simulink model "FirstItem"  (R2022b)
settings: Solver=ode4  StartTime=0.0  StopTime=45  FixedStep=0.01  RelTol=1e-3
values from neighbouring files (symbols this model uses):
  Ka = 4.5    [Item1.m]
  Kdc = 1.1    [Item1.m]
  Ki = 14.3    [Item1.m]
  Kr = -0.37    [Item1.m]
  l_MO = 80*d2r    (= 1.3962634016)    [Item1.m]
  l_TO = -2.5*d2r    (= -0.0436332312999)    [Item1.m]
  V_T = 600    [Item1.m]
  X_MO = 2000    [Item1.m]
  X_TO = 100    [Item1.m]
  Z_MO = 0    [Item1.m]
  Z_TO = 20000    [Item1.m]
libraries: simulink x1
settings Model: Creator=lagruni  LastModifiedBy=lagruni

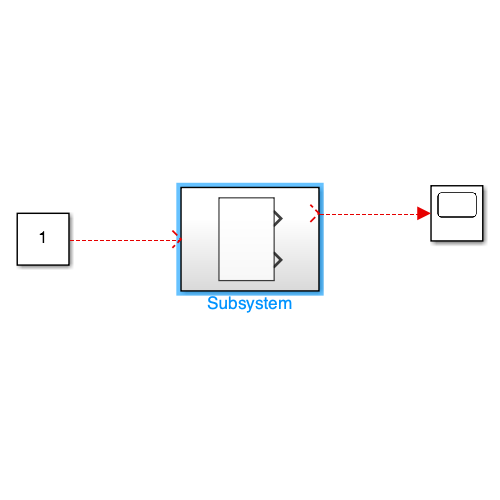
[thumbnail: Simulink's stored preview of the top-level diagram]
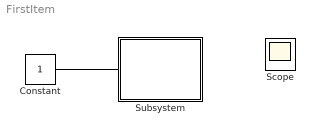
== system FirstItem ==
  Constant : Constant
  Scope : Scope
  Subsystem : Subsystem
  wires:
  Constant/1 -> ?
  ? -> Scope/1

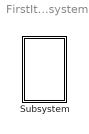
== system FirstItem/Subsystem ==
  Subsystem : Subsystem

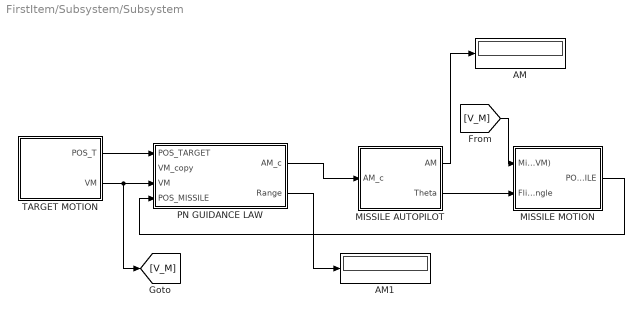
== system FirstItem/Subsystem/Subsystem ==
  AM : Display
      settings: Format=bank
  AM1 : Display
      settings: Format=bank
  MISSILE AUTOPILOT : Subsystem
  MISSILE MOTION : Subsystem
  PN GUIDANCE LAW : Subsystem
  TARGET MOTION : Subsystem
  wires:
  TARGET MOTION/1(POS_T) -> PN GUIDANCE LAW/1(POS_TARGET)
  TARGET MOTION/2(VM) -> [V_M], PN GUIDANCE LAW/3(VM)
  [V_M] -> MISSILE MOTION/1(Missile speed (VM))
  MISSILE MOTION/1(POS_MISSILE) -> PN GUIDANCE LAW/4(POS_MISSILE)
  PN GUIDANCE LAW/1(AM_c) -> MISSILE AUTOPILOT/1(AM_c)
  MISSILE AUTOPILOT/2(Theta) -> MISSILE MOTION/2(Flight path angle)
  MISSILE AUTOPILOT/1(AM) -> AM/1
  PN GUIDANCE LAW/2(Range) -> AM1/1

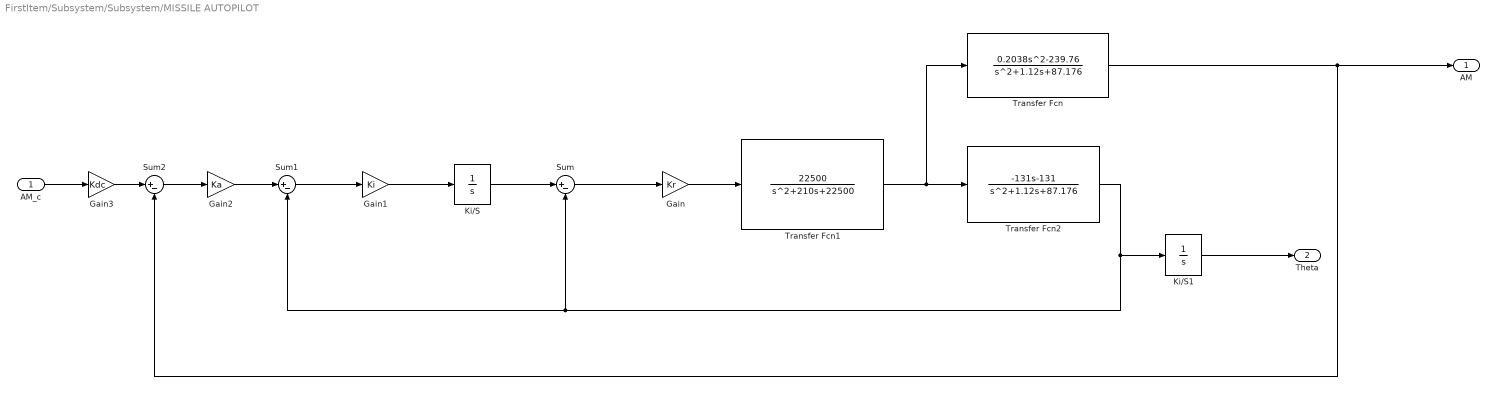
== system FirstItem/Subsystem/Subsystem/MISSILE AUTOPILOT ==
  AM_c : Inport
  Gain : Gain  Gain=Kr
  Gain1 : Gain  Gain=Ki
  Gain2 : Gain  Gain=Ka
  Gain3 : Gain  Gain=Kdc
  Ki/S : Integrator
  Ki/S1 : Integrator  InitialCondition=l_MO
  Sum : Sum  Inputs=|+-
  Sum1 : Sum  Inputs=|+-
  Sum2 : Sum  Inputs=|+-
  Transfer Fcn : TransferFcn  Numerator=[0.2038 0 -239.76]  Denominator=[1 1.12 87.176]
  Transfer Fcn1 : TransferFcn  Numerator=[22500]  Denominator=[1 210 22500]
  Transfer Fcn2 : TransferFcn  Numerator=[-131 -131]  Denominator=[1 1.12 87.176]
  AM : Outport
  Theta : Outport  Port=2
  wires:
  AM_c/1 -> Gain3/1
  Sum/1 -> Gain/1
  Transfer Fcn2/1 -> Ki/S1/1, Sum/2, Sum1/2
  Transfer Fcn1/1 -> Transfer Fcn/1, Transfer Fcn2/1
  Ki/S1/1 -> Theta/1
  Gain/1 -> Transfer Fcn1/1
  Sum1/1 -> Gain1/1
  Ki/S/1 -> Sum/1
  Gain2/1 -> Sum1/1
  Sum2/1 -> Gain2/1
  Gain3/1 -> Sum2/1
  Gain1/1 -> Ki/S/1
  Transfer Fcn/1 -> AM/1, Sum2/2

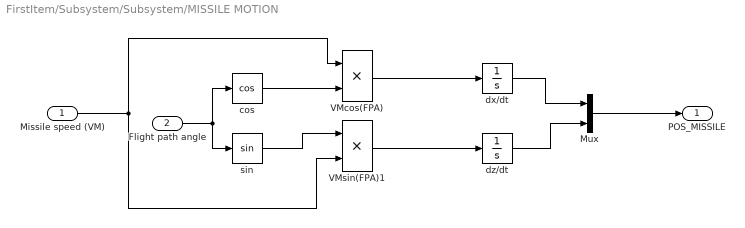
== system FirstItem/Subsystem/Subsystem/MISSILE MOTION ==
  Missile speed (VM) : Inport
  Flight path angle : Inport  Port=2
  Mux : Mux  Inputs=2
  VMcos(FPA) : Product
  VMsin(FPA)1 : Product
  cos : Trigonometry  Operator=cos
  dx/dt : Integrator  InitialCondition=X_MO
  dz/dt : Integrator  InitialCondition=Z_MO
  sin : Trigonometry
  POS_MISSILE : Outport
  wires:
  Mux/1 -> POS_MISSILE/1
  cos/1 -> VMcos(FPA)/2
  dz/dt/1 -> Mux/2
  Missile speed (VM)/1 -> VMsin(FPA)1/2, VMcos(FPA)/1
  sin/1 -> VMsin(FPA)1/1
  VMsin(FPA)1/1 -> dz/dt/1
  dx/dt/1 -> Mux/1
  VMcos(FPA)/1 -> dx/dt/1
  Flight path angle/1 -> sin/1, cos/1

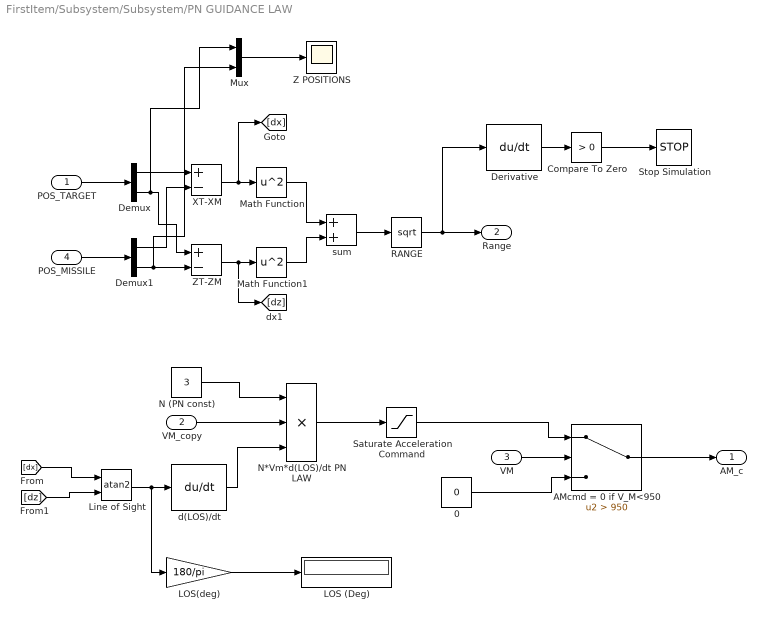
== system FirstItem/Subsystem/Subsystem/PN GUIDANCE LAW ==
  POS_TARGET : Inport
  VM_copy : Inport  Port=2
  VM : Inport  Port=3
  POS_MISSILE : Inport  Port=4
  0 : Constant  Value=0
  AMcmd = 0 if V_M<950 : Switch  Criteria=u2 > Threshold  Threshold=950  SaturateOnIntegerOverflow=off  InputSameDT=off
  Compare To Zero : simulink/Logic and Bit Operations/Compare To Zero  relop=>  OutDataTypeStr=boolean
  Demux : Demux  Outputs=2
  Demux1 : Demux  Outputs=2
  Derivative : Derivative
  LOS (Deg) : Display
  LOS(deg) : Gain  Gain=180/pi
  Line of Sight : Trigonometry  Operator=atan2
  Math Function : Math  Operator=square
  Math Function1 : Math  Operator=square
  Mux : Mux  Inputs=2
  N (PN const) : Constant  Value=3
  N*Vm*d(LOS)/dt PN LAW : Product  Inputs=3
  RANGE : Sqrt
  Saturate Acceleration Command : Saturate  UpperLimit=0  LowerLimit=-0.10
  Stop Simulation : Stop
  XT-XM : Sum  Inputs=+-
  Z POSITIONS : Scope
  ZT-ZM : Sum  Inputs=+-
  d(LOS)/dt : Derivative
  sum : Sum
  AM_c : Outport
  Range : Outport  Port=2
  wires:
  Saturate Acceleration Command/1 -> AMcmd = 0 if V_M<950/1
  LOS(deg)/1 -> LOS (Deg)/1
  RANGE/1 -> Range/1, Derivative/1
  VM_copy/1 -> N*Vm*d(LOS)/dt PN LAW/2
  POS_TARGET/1 -> Demux/1
  N (PN const)/1 -> N*Vm*d(LOS)/dt PN LAW/1
  VM/1 -> AMcmd = 0 if V_M<950/2
  AMcmd = 0 if V_M<950/1 -> AM_c/1
  POS_MISSILE/1 -> Demux1/1
  N*Vm*d(LOS)/dt PN LAW/1 -> Saturate Acceleration Command/1
  Mux/1 -> Z POSITIONS/1
  Demux1/1 -> XT-XM/2
  Math Function1/1 -> sum/2
  [dz] -> Line of Sight/2
  sum/1 -> RANGE/1
  Demux/1 -> XT-XM/1
  ZT-ZM/1 -> [dz], Math Function1/1
  0/1 -> AMcmd = 0 if V_M<950/3
  Compare To Zero/1 -> Stop Simulation/1
  Demux1/2 -> Mux/2, ZT-ZM/2
  Demux/2 -> Mux/1, ZT-ZM/1
  XT-XM/1 -> [dx], Math Function/1
  Derivative/1 -> Compare To Zero/1
  Line of Sight/1 -> LOS(deg)/1, d(LOS)/dt/1
  Math Function/1 -> sum/1
  d(LOS)/dt/1 -> N*Vm*d(LOS)/dt PN LAW/3
  [dx] -> Line of Sight/1

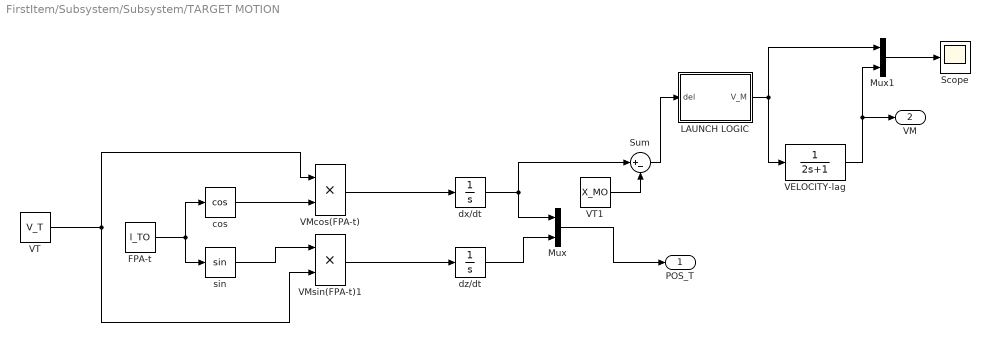
== system FirstItem/Subsystem/Subsystem/TARGET MOTION ==
  FPA-t : Constant  Value=l_TO
  LAUNCH LOGIC : MATLAB Function  TreatAsAtomicUnit=on
  Mux : Mux  Inputs=2
  Mux1 : Mux  Inputs=2
  Scope : Scope
  Sum : Sum  Inputs=|+-
  VELOCITY-lag : TransferFcn  Denominator=[2 1]
  VMcos(FPA-t) : Product
  VMsin(FPA-t)1 : Product
  VT : Constant  Value=V_T
  VT1 : Constant  Value=X_MO
  cos : Trigonometry  Operator=cos
  dx/dt : Integrator  InitialCondition=X_TO
  dz/dt : Integrator  InitialCondition=Z_TO
  sin : Trigonometry
  POS_T : Outport
  VM : Outport  Port=2
  wires:
  Mux1/1 -> Scope/1
  VT1/1 -> Sum/2
  VMcos(FPA-t)/1 -> dx/dt/1
  cos/1 -> VMcos(FPA-t)/2
  VMsin(FPA-t)1/1 -> dz/dt/1
  LAUNCH LOGIC/1(V_M) -> VELOCITY-lag/1, Mux1/1
  dz/dt/1 -> Mux/2
  Sum/1 -> LAUNCH LOGIC/1(del)
  Mux/1 -> POS_T/1
  FPA-t/1 -> sin/1, cos/1
  VELOCITY-lag/1 -> VM/1, Mux1/2
  dx/dt/1 -> Mux/1, Sum/1
  sin/1 -> VMsin(FPA-t)1/1
  VT/1 -> VMsin(FPA-t)1/2, VMcos(FPA-t)/1

== matlab function FirstItem/Subsystem/Subsystem/TARGET MOTION/LAUNCH LOGIC ==
  settings: updateMethod=DISCRETE
  data: del input; V_M output
function V_M = fcn(del)
%#codegen
persistent f
persistent Vel

if isempty(f) 
    f = 0;
end
if isempty(Vel)
    Vel = 0;
end
if f == 0 && del > -200
    f = 1;
    Vel = 1021; %missile speed
end

V_M = Vel;
